simulink model "BLDCMachine_HystController_TorqueControl"  (R2018b)
settings: Solver=ode4  StartTime=0.0  StopTime=10  FixedStep=0.000005  MaxStep=1e-4  RelTol=1e-5
libraries: powerlib x16, dsparch4 x8, simulink x2
settings Model: Creator=uidp4945  LastModifiedBy=axint
settings SolverCC: AlgebraicLoopSolver=LineSearch
settings SFSimCC: SimUseLocalCustomCode=off
settings RTWCC: RTWUseLocalCustomCode=off

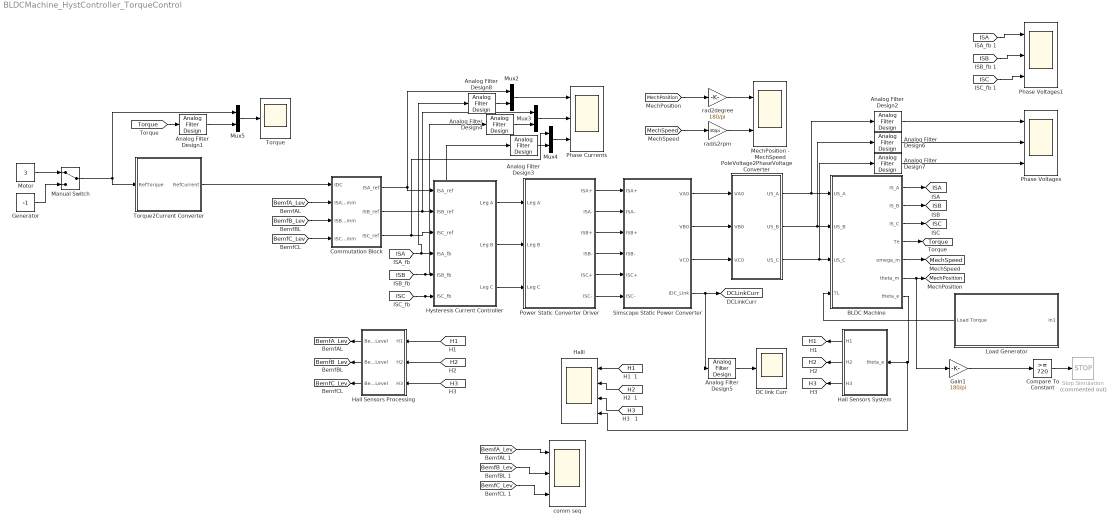
== system BLDCMachine_HystController_TorqueControl ==
  Analog Filter Design1 : dsparch4/Analog Filter Design  method=Butterworth  filttype=Lowpass  N=2  Wlo=500  Whi=80  Rp=2  Rs=40
  Analog Filter Design{2..8} (7 alike) : dsparch4/Analog Filter Design  method=Butterworth  filttype=Lowpass  N=2  Wlo=2000  Whi=80  Rp=2  Rs=40
  BLDC Machine : Subsystem  mask{Rs=0.2, Ls=0.0085*1e0, Flux=0.175, J=0.089, D=5e-5, p=4}
      mask prompts: Rs "Stator resistance [ohm]"; Ls "Equivalent stator inductance [H]"; Flux "Rotor magnetic flux [Wb]"; J "Moment of inertia [Kgm^2]"; D "Viscous coefficient [Nm s/rad]"; p "Number of pole pairs"
  Commutation Block : Subsystem
  Compare To Constant : simulink/Logic and Bit Operations/Compare To Constant  relop=>=  const=720  OutDataTypeStr=boolean
  DC link Curr : Scope
  Gain1 : Gain  Gain=180/pi
  Generator : Constant  Value=-1
  Hall Sensors Processing : Subsystem
  Hall Sensors System : Subsystem
  Halll : Scope  NumInputPorts=4
  Hysteresis Current Controller : Subsystem  mask{h=0.01}
      mask prompts: h "Hysteresis value [A]"
  Load Generator : Subsystem
  Manual Switch : ManualSwitch
  MechPosition - MechSpeed : Scope  NumInputPorts=2
  Motor : Constant  Value=3
  Mux{2..5} (4 alike) : Mux  Inputs=2
  Phase Currents : Scope  NumInputPorts=3
  Phase Voltages : Scope  NumInputPorts=3
  Phase Voltages1 : Scope  NumInputPorts=3
  PoleVoltage2PhaseVoltage Converter : Subsystem
  Power Static Converter Driver : Subsystem
  "Simscape Static Power Converter " : Subsystem  mask{VDC=500}
      mask prompts: VDC "Voltage DC Link"
  Stop Simulation : Stop  Commented=on
  "Torque " : Scope
  Torque2Current Converter : Subsystem  mask{Flux=0.175, p=4}
      mask prompts: Flux "Rotor Magnetic Flux [Wb]"; p "Number of pole pairs"
  comm seq : Scope  NumInputPorts=3
  rad/s2rpm : Gain  Gain=30/pi
  rad2degree : Gain  Gain=180/pi
  tag scope: BemfA_Lev=global, BemfB_Lev=global, BemfC_Lev=global, DCLinkCurr=global, H1=global, H2=global, H3=global, ISA=global, ISB=global, ISC=global, MechPosition=global, MechSpeed=global, Torque=global
  wires:
  "Simscape Static Power Converter "/1("VA0 ") -> PoleVoltage2PhaseVoltage Converter/1(VA0)
  "Simscape Static Power Converter "/2("VB0 ") -> PoleVoltage2PhaseVoltage Converter/2(VB0)
  "Simscape Static Power Converter "/3("VC0 ") -> PoleVoltage2PhaseVoltage Converter/3(VC0)
  PoleVoltage2PhaseVoltage Converter/1(US_A) -> Analog Filter Design2/1, BLDC Machine/1(US_A)
  PoleVoltage2PhaseVoltage Converter/2(US_B) -> Analog Filter Design6/1, BLDC Machine/2(US_B)
  PoleVoltage2PhaseVoltage Converter/3(US_C) -> Analog Filter Design7/1, BLDC Machine/3(US_C)
  Load Generator/1("Load Torque ") -> BLDC Machine/4(TL)
  BLDC Machine/1(IS_A) -> [ISA]
  BLDC Machine/2(IS_B) -> [ISB]
  BLDC Machine/3(IS_C) -> [ISC]
  BLDC Machine/5("omega_m  ") -> [MechSpeed]
  BLDC Machine/6("theta_m ") -> Gain1/1, [MechPosition]
  Hall Sensors System/1(H1) -> [H1]
  Hall Sensors System/2(H2) -> [H2]
  Hall Sensors System/3(H3) -> [H3]
  [H1] -> Hall Sensors Processing/1(H1)
  [H2] -> Hall Sensors Processing/2(H2)
  [H3] -> Hall Sensors Processing/3(H3)
  Hall Sensors Processing/1(BemfA Level) -> [BemfA_Lev]
  Hall Sensors Processing/2(BemfB Level) -> [BemfB_Lev]
  Hall Sensors Processing/3(BemfC Level) -> [BemfC_Lev]
  Power Static Converter Driver/2(ISA-) -> "Simscape Static Power Converter "/2(ISA-)
  Power Static Converter Driver/4(ISB-) -> "Simscape Static Power Converter "/4(ISB-)
  Power Static Converter Driver/6(ISC-) -> "Simscape Static Power Converter "/6(ISC-)
  Power Static Converter Driver/1(ISA+) -> "Simscape Static Power Converter "/1(ISA+)
  Power Static Converter Driver/3(ISB+) -> "Simscape Static Power Converter "/3(ISB+)
  Power Static Converter Driver/5(ISC+) -> "Simscape Static Power Converter "/5(ISC+)
  Hysteresis Current Controller/1(Leg A) -> Power Static Converter Driver/1(Leg A)
  Commutation Block/2(ISB_ref) -> Mux3/1, Hysteresis Current Controller/2(ISB_ref)
  Commutation Block/3(ISC_ref) -> Hysteresis Current Controller/3(ISC_ref), Mux4/1
  [ISB] -> Analog Filter Design4/1, Hysteresis Current Controller/5(ISB_fb)
  [ISC] -> Analog Filter Design3/1, Hysteresis Current Controller/6(ISC_fb)
  Hysteresis Current Controller/2(Leg B) -> Power Static Converter Driver/2(Leg B)
  Hysteresis Current Controller/3(Leg C) -> Power Static Converter Driver/3(Leg C)
  Mux2/1 -> Phase Currents/1
  Commutation Block/1(ISA_ref) -> Hysteresis Current Controller/1(ISA_ref), Mux2/1
  Mux3/1 -> Phase Currents/2
  Mux4/1 -> Phase Currents/3
  BLDC Machine/4(Te) -> [Torque]
  Mux5/1 -> "Torque "/1
  [Torque] -> Analog Filter Design1/1
  "Simscape Static Power Converter "/4(IDC_Link) -> Analog Filter Design5/1, [DCLinkCurr]
  [MechPosition] -> rad2degree/1
  [MechSpeed] -> rad/s2rpm/1
  rad2degree/1 -> MechPosition - MechSpeed/1
  rad/s2rpm/1 -> MechPosition - MechSpeed/2
  Analog Filter Design1/1 -> Mux5/2
  Torque2Current Converter/1(RefCurrent) -> Commutation Block/1(IDC)
  Analog Filter Design2/1 -> Phase Voltages/1
  Manual Switch/1 -> Mux5/1, Torque2Current Converter/1(RefTorque)
  Analog Filter Design3/1 -> Mux4/2
  Analog Filter Design4/1 -> Mux3/2
  Analog Filter Design6/1 -> Phase Voltages/2
  Analog Filter Design7/1 -> Phase Voltages/3
  [ISA] -> Analog Filter Design8/1, Hysteresis Current Controller/4(ISA_fb)
  [BemfA_Lev] -> Commutation Block/2(ISA comm)
  [BemfB_Lev] -> Commutation Block/3(ISB comm)
  [BemfC_Lev] -> Commutation Block/4(ISC comm)
  Gain1/1 -> Compare To Constant/1
  Compare To Constant/1 -> Stop Simulation/1
  Generator/1 -> Manual Switch/2
  Motor/1 -> Manual Switch/1
  Analog Filter Design5/1 -> DC link Curr/1
  [H1] -> Halll/1
  [H2] -> Halll/2
  [H3] -> Halll/3
  BLDC Machine/7(theta_e) -> Halll/4, Hall Sensors System/1(theta_e)
  [ISA] -> Phase Voltages1/1
  [ISB] -> Phase Voltages1/2
  [ISC] -> Phase Voltages1/3
  Analog Filter Design8/1 -> Mux2/2
  [BemfA_Lev] -> comm seq/1
  [BemfB_Lev] -> comm seq/2
  [BemfC_Lev] -> comm seq/3

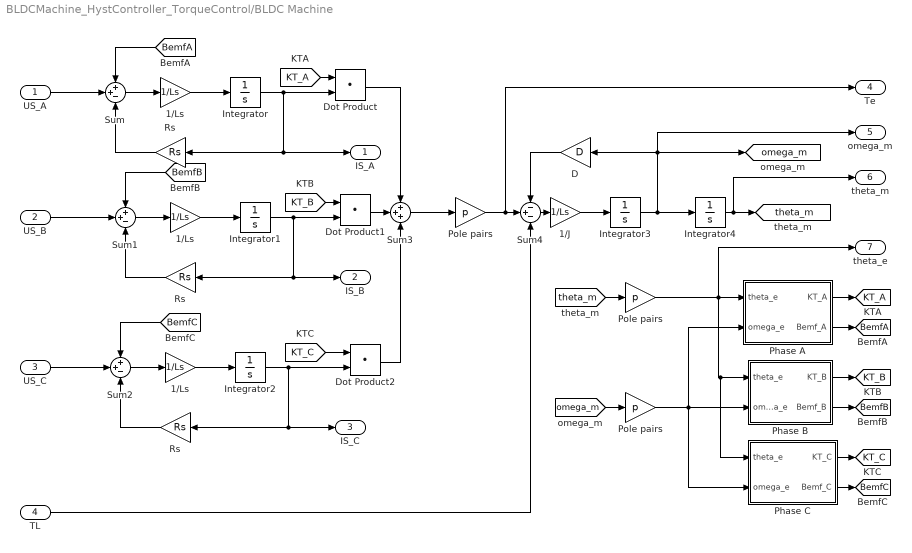
== system BLDCMachine_HystController_TorqueControl/BLDC Machine ==
  US_A : Inport
  US_B : Inport  Port=2
  US_C : Inport  Port=3
  TL : Inport  Port=4
  1/J : Gain  Gain=1/Ls
  1/Ls : Gain  Gain=1/Ls
  "1/Ls " : Gain  Gain=1/Ls
  "1/Ls  " : Gain  Gain=1/Ls
  D : Gain  Gain=D
  Dot Product : DotProduct  InputSameDT=on  OutDataTypeStr=Inherit: Inherit via internal rule
  Dot Product1 : DotProduct  InputSameDT=on  OutDataTypeStr=Inherit: Inherit via internal rule
  Dot Product2 : DotProduct  InputSameDT=on  OutDataTypeStr=Inherit: Inherit via internal rule
  Integrator{,1..4} (5 alike) : Integrator
  Phase A : Subsystem
  Phase B : Subsystem
  Phase C : Subsystem
  Pole pairs : Gain  Gain=p
  "Pole pairs  " : Gain  Gain=p
  "Pole pairs   " : Gain  Gain=p
  Rs : Gain  Gain=Rs
  "Rs " : Gain  Gain=Rs
  "Rs  " : Gain  Gain=Rs
  Sum : Sum  Inputs=++-
  Sum1 : Sum  Inputs=++-
  Sum2 : Sum  Inputs=++-
  Sum3 : Sum  Inputs=+++
  Sum4 : Sum  Inputs=-+-
  IS_A : Outport
  IS_B : Outport  Port=2
  IS_C : Outport  Port=3
  Te : Outport  Port=4
  "omega_m  " : Outport  Port=5
  "theta_m " : Outport  Port=6
  theta_e : Outport  Port=7
  tag scope: BemfA=global, BemfB=global, BemfC=global, KT_A=global, KT_B=global, KT_C=global, omega_m=global, theta_m=global
  wires:
  [KT_C] -> Dot Product2/1
  Sum4/1 -> 1/J/1
  Dot Product1/1 -> Sum3/2
  Phase B/1(KT_B) -> [KT_B]
  Phase A/1(KT_A) -> [KT_A]
  Dot Product2/1 -> Sum3/3
  Dot Product/1 -> Sum3/1
  Phase C/1(KT_C) -> [KT_C]
  Integrator/1 -> Dot Product/2, IS_A/1, Rs/1
  Integrator4/1 -> [theta_m], "theta_m "/1
  Pole pairs/1 -> Phase C/2(omega_e), Phase B/2(omega_e), Phase A/2(omega_e)
  "Pole pairs  "/1 -> theta_e/1, Phase C/1(theta_e), Phase B/1(theta_e), Phase A/1(theta_e)
  D/1 -> Sum4/1
  [BemfC] -> Sum2/1
  Sum2/1 -> "1/Ls  "/1
  "1/Ls  "/1 -> Integrator2/1
  Integrator2/1 -> Dot Product2/2, IS_C/1, "Rs  "/1
  US_C/1 -> Sum2/2
  "Rs  "/1 -> Sum2/3
  Phase B/2(Bemf_B) -> [BemfB]
  Phase C/2(Bemf_C) -> [BemfC]
  Integrator1/1 -> Dot Product1/2, IS_B/1, "Rs "/1
  1/J/1 -> Integrator3/1
  [omega_m] -> Pole pairs/1
  [KT_B] -> Dot Product1/1
  Phase A/2(Bemf_A) -> [BemfA]
  TL/1 -> Sum4/3
  [KT_A] -> Dot Product/1
  [BemfA] -> Sum/1
  US_A/1 -> Sum/2
  Rs/1 -> Sum/3
  [theta_m] -> "Pole pairs  "/1
  Integrator3/1 -> "omega_m  "/1, D/1, [omega_m], Integrator4/1
  1/Ls/1 -> Integrator/1
  "1/Ls "/1 -> Integrator1/1
  Sum1/1 -> "1/Ls "/1
  US_B/1 -> Sum1/2
  "Rs "/1 -> Sum1/3
  [BemfB] -> Sum1/1
  Sum/1 -> 1/Ls/1
  Sum3/1 -> "Pole pairs   "/1
  "Pole pairs   "/1 -> Te/1, Sum4/2

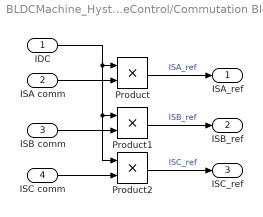
== system BLDCMachine_HystController_TorqueControl/Commutation Block ==
  IDC : Inport
  ISA comm : Inport  Port=2
  ISB comm : Inport  Port=3
  ISC comm : Inport  Port=4
  Product : Product
  Product1 : Product
  Product2 : Product
  ISA_ref : Outport
  ISB_ref : Outport  Port=2
  ISC_ref : Outport  Port=3
  wires:
  ISC comm/1 -> Product2/2
  Product/1 -> ISA_ref/1  "ISA_ref"
  IDC/1 -> Product2/1, Product1/1, Product/1
  ISB comm/1 -> Product1/2
  ISA comm/1 -> Product/2
  Product2/1 -> ISC_ref/1  "ISC_ref"
  Product1/1 -> ISB_ref/1  "ISB_ref"

== system BLDCMachine_HystController_TorqueControl/Hall Sensors Processing ==
  H1 : Inport
  H2 : Inport  Port=2
  H3 : Inport  Port=3
  BemfA Saturation Level : Subsystem
  BemfB Saturation Level : Subsystem
  BemfC Saturation Level : Subsystem
  BemfA Level : Outport
  BemfB Level : Outport  Port=2
  BemfC Level : Outport  Port=3
  wires:
  BemfB Saturation Level/1("BenfB Level ") -> BemfB Level/1
  H2/1 -> BemfC Saturation Level/1(H2), BemfB Saturation Level/2(H2)
  H1/1 -> BemfB Saturation Level/1(H1), BemfA Saturation Level/1(H1)
  BemfC Saturation Level/1("BenfC Level ") -> BemfC Level/1
  BemfA Saturation Level/1("BenfA Level ") -> BemfA Level/1
  H3/1 -> BemfC Saturation Level/2(H3), BemfA Saturation Level/2(H3)

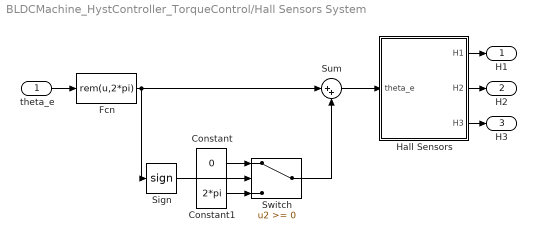
== system BLDCMachine_HystController_TorqueControl/Hall Sensors System ==
  theta_e : Inport
  Constant : Constant  Value=0
  Constant1 : Constant  Value=2*pi
  Fcn : Fcn  Expr=rem(u,2*pi)
  Hall Sensors : Subsystem
  Sign : Signum
  Sum : Sum  Inputs=|++
  Switch : Switch
  H1 : Outport
  H2 : Outport  Port=2
  H3 : Outport  Port=3
  wires:
  Hall Sensors/3("H3 ") -> H3/1
  Hall Sensors/1("H1 ") -> H1/1
  Hall Sensors/2("H2 ") -> H2/1
  theta_e/1 -> Fcn/1
  Fcn/1 -> Sum/1, Sign/1
  Sign/1 -> Switch/2
  Constant1/1 -> Switch/3
  Switch/1 -> Sum/2
  Sum/1 -> Hall Sensors/1(theta_e)
  Constant/1 -> Switch/1

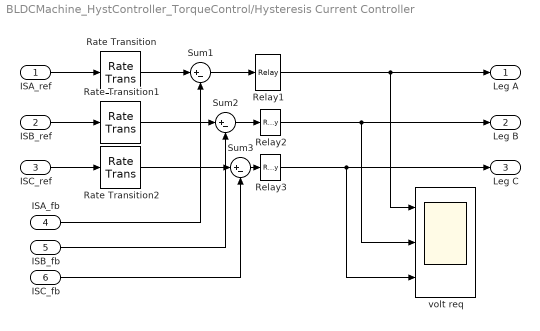
== system BLDCMachine_HystController_TorqueControl/Hysteresis Current Controller ==
  ISA_ref : Inport
  ISB_ref : Inport  Port=2
  ISC_ref : Inport  Port=3
  ISA_fb : Inport  Port=4
  ISB_fb : Inport  Port=5
  ISC_fb : Inport  Port=6
  Rate Transition : RateTransition  OutPortSampleTime=0.000025
  Rate Transition1 : RateTransition  OutPortSampleTime=0.000025
  Rate Transition2 : RateTransition  OutPortSampleTime=0.000025
  Relay1 : Relay  OnSwitchValue=h/2  OffSwitchValue=-h/2  OffOutputValue=-1
  Relay2 : Relay  OnSwitchValue=h/2  OffSwitchValue=-h/2  OffOutputValue=-1
  Relay3 : Relay  OnSwitchValue=h/2  OffSwitchValue=-h/2  OffOutputValue=-1
  Sum1 : Sum  Inputs=|+-
  Sum2 : Sum  Inputs=|+-
  Sum3 : Sum  Inputs=|+-
  volt req : Scope  NumInputPorts=3
  Leg A : Outport
  Leg B : Outport  Port=2
  Leg C : Outport  Port=3
  wires:
  ISC_fb/1 -> Sum3/2
  ISA_fb/1 -> Sum1/2
  Sum3/1 -> Relay3/1
  ISA_ref/1 -> Rate Transition/1
  Sum2/1 -> Relay2/1
  ISB_fb/1 -> Sum2/2
  Relay1/1 -> volt req/1, Leg A/1
  Relay2/1 -> volt req/2, Leg B/1
  Sum1/1 -> Relay1/1
  ISC_ref/1 -> Rate Transition2/1
  Relay3/1 -> volt req/3, Leg C/1
  ISB_ref/1 -> Rate Transition1/1
  Rate Transition/1 -> Sum1/1
  Rate Transition1/1 -> Sum2/1
  Rate Transition2/1 -> Sum3/1

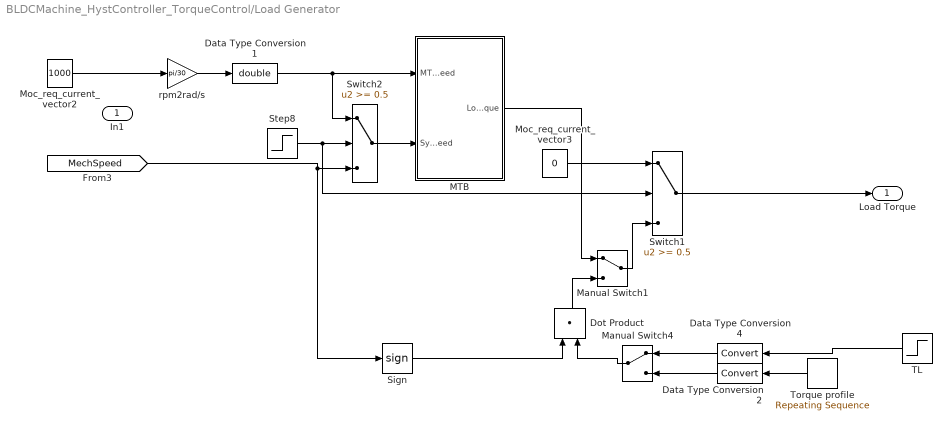
== system BLDCMachine_HystController_TorqueControl/Load Generator ==
  In1 : Inport
  Data Type Conversion1 : DataTypeConversion  OutDataTypeStr=double
  Data Type Conversion2 : DataTypeConversion
  Data Type Conversion4 : DataTypeConversion
  Dot Product : DotProduct  InputSameDT=on  OutDataTypeStr=Inherit: Inherit via internal rule
  MTB : Subsystem
  Manual Switch1 : ManualSwitch
  Manual Switch4 : ManualSwitch
  Moc_req_current_vector2 : Constant  Value=1000  OutDataTypeStr=Inherit: Inherit via back propagation
  Moc_req_current_vector3 : Constant  Value=0  OutDataTypeStr=Inherit: Inherit via back propagation
  Sign : Signum
  Step8 : Step  Time=0  Before=1  After=0  SampleTime=0
  Switch1 : Switch  Threshold=0.5
  Switch2 : Switch  Threshold=0.5
  TL : Step  Time=0.5  After=10*0.5  SampleTime=0
  Torque profile : simulink/Sources/Repeating Sequence  rep_seq_t="[0 0.12    0.24   0.48 ]"  rep_seq_y="[1   1     -1 -1]*0"
  rpm2rad/s : Gain  Gain=pi/30
  "Load Torque " : Outport
  wires:
  Switch2/1 -> MTB/2(Sys_Speed)
  Manual Switch1/1 -> Switch1/3
  Step8/1 -> Switch1/2, Switch2/2
  MTB/1(Load_Torque) -> Manual Switch1/1
  Moc_req_current_vector3/1 -> Switch1/1
  Dot Product/1 -> Manual Switch1/2
  Sign/1 -> Dot Product/1
  Manual Switch4/1 -> Dot Product/2
  Torque profile/1 -> Data Type Conversion2/1
  Data Type Conversion2/1 -> Manual Switch4/2
  Data Type Conversion4/1 -> Manual Switch4/1
  Moc_req_current_vector2/1 -> rpm2rad/s/1
  Data Type Conversion1/1 -> Switch2/1, MTB/1(MTB_Speed)
  TL/1 -> Data Type Conversion4/1
  rpm2rad/s/1 -> Data Type Conversion1/1
  [MechSpeed] -> Switch2/3, Sign/1
  Switch1/1 -> "Load Torque "/1

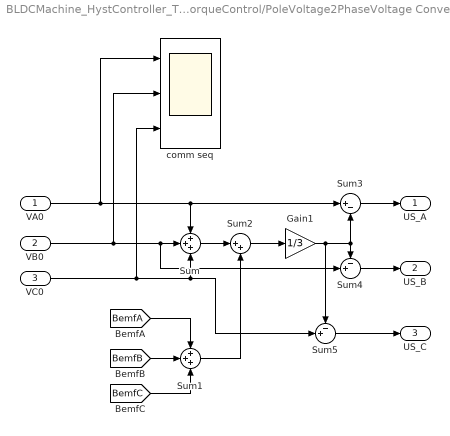
== system BLDCMachine_HystController_TorqueControl/PoleVoltage2PhaseVoltage Converter ==
  VA0 : Inport
  VB0 : Inport  Port=2
  VC0 : Inport  Port=3
  Gain1 : Gain  Gain=1/3
  Sum : Sum  Inputs=+++
  Sum1 : Sum  Inputs=+++
  Sum2 : Sum  Inputs=|++
  Sum3 : Sum  Inputs=|+-
  Sum4 : Sum  Inputs=-+|
  Sum5 : Sum  Inputs=-+|
  comm seq : Scope  NumInputPorts=3
  US_A : Outport
  US_B : Outport  Port=2
  US_C : Outport  Port=3
  wires:
  VB0/1 -> comm seq/2, Sum4/2, Sum/2
  [BemfC] -> Sum1/3
  [BemfA] -> Sum1/1
  [BemfB] -> Sum1/2
  VC0/1 -> comm seq/3, Sum5/2, Sum/3
  Sum3/1 -> US_A/1
  VA0/1 -> comm seq/1, Sum3/1, Sum/1
  Sum1/1 -> Sum2/2
  Sum4/1 -> US_B/1
  Sum/1 -> Sum2/1
  Sum2/1 -> Gain1/1
  Gain1/1 -> Sum4/1, Sum3/2, Sum5/1
  Sum5/1 -> US_C/1

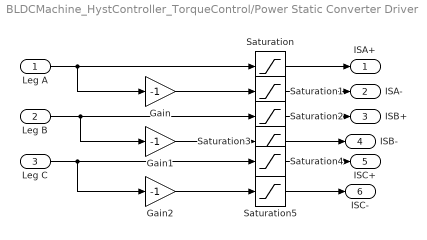
== system BLDCMachine_HystController_TorqueControl/Power Static Converter Driver ==
  Leg A : Inport
  Leg B : Inport  Port=2
  Leg C : Inport  Port=3
  Gain : Gain  Gain=-1
  Gain1 : Gain  Gain=-1
  Gain2 : Gain  Gain=-1
  Saturation{,1..5} (6 alike) : Saturate  UpperLimit=1  LowerLimit=0
  ISA+ : Outport
  ISA- : Outport  Port=2
  ISB+ : Outport  Port=3
  ISB- : Outport  Port=4
  ISC+ : Outport  Port=5
  ISC- : Outport  Port=6
  wires:
  Gain/1 -> Saturation1/1
  Gain1/1 -> Saturation3/1
  Leg C/1 -> Gain2/1, Saturation4/1
  Leg A/1 -> Gain/1, Saturation/1
  Gain2/1 -> Saturation5/1
  Leg B/1 -> Gain1/1, Saturation2/1
  Saturation/1 -> ISA+/1
  Saturation1/1 -> ISA-/1
  Saturation2/1 -> ISB+/1
  Saturation3/1 -> ISB-/1
  Saturation4/1 -> ISC+/1
  Saturation5/1 -> ISC-/1

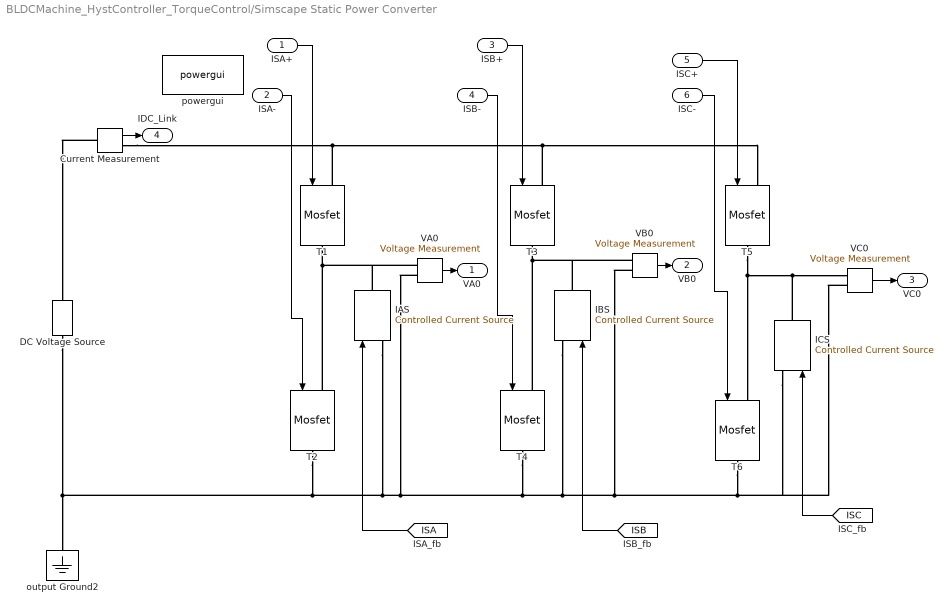
== system BLDCMachine_HystController_TorqueControl/Simscape Static Power Converter  ==
  ISA+ : Inport
  ISA- : Inport  Port=2
  ISB+ : Inport  Port=3
  ISB- : Inport  Port=4
  ISC+ : Inport  Port=5
  ISC- : Inport  Port=6
  Current Measurement : powerlib/Measurements/Current Measurement  PhasorSimulation=off  OutputType=Complex  PSBequivalent=0
      settings: SourceProductName=Simscape Electrical
  DC Voltage Source : powerlib/Electrical Sources/DC Voltage Source  Amplitude=VDC  Measurements=None
      settings: SourceProductName=Simscape Electrical
  IAS : powerlib/Electrical Sources/Controlled Current Source  Initialize=on  Source_Type=DC  Amplitude=0  Phase=0  Frequency=0  Measurements=None
      settings: SourceProductName=Simscape Electrical
  IBS : powerlib/Electrical Sources/Controlled Current Source  Initialize=on  Source_Type=DC  Amplitude=0  Phase=0  Frequency=0  Measurements=None
      settings: SourceProductName=Simscape Electrical
  ICS : powerlib/Electrical Sources/Controlled Current Source  Initialize=on  Source_Type=DC  Amplitude=0  Phase=0  Frequency=0  Measurements=None
      settings: SourceProductName=Simscape Electrical
  T{1..6} (6 alike) : powerlib/Power Electronics/Mosfet  Ron=0.1  Lon=0  Rd=0.01  Vfd=0  IC=0  Rs=1e5  Cs=inf  Measurements=off
      settings: SourceProductName=Simscape Electrical
  VA0 : powerlib/Measurements/Voltage Measurement  PhasorSimulation=off  OutputType=Complex  PSBequivalent=0
      settings: SourceProductName=Simscape Electrical
  VB0 : powerlib/Measurements/Voltage Measurement  PhasorSimulation=off  OutputType=Complex  PSBequivalent=0
      settings: SourceProductName=Simscape Electrical
  VC0 : powerlib/Measurements/Voltage Measurement  PhasorSimulation=off  OutputType=Complex  PSBequivalent=0
      settings: SourceProductName=Simscape Electrical
  output Ground2 : powerlib/Elements/Ground  LConnTagsString=a
      settings: SourceProductName=Simscape Electrical
  powergui : powerlib/powergui  Priority=1  SimulationMode=Continuous  SampleTime=0.0001  frequency=60  Iterations=50  frequencyindice=0  Pbase=100e6  ErrMax=1e-4  UnitsV=kV  UnitsW=MW  buscounter=0  FunctionMessages=off  echomessages=off  EnableUseOfTLC=off  CurrentSourceSwitches=off  DisableSnubberDevices=off  DisableRonSwitches=off  DisableVfSwitches=off  DisplayEquations=off  SolverType=Tustin/Backward Euler (TBE)  Interpol=off  ExternalGateDelay=off  methode=off  Ts=100  x0status=blocks  SPID=on  SwTol=0  HookPort=off  RestoreLinks=warning  ResistiveCurrentMeasurement=off  Frange=[0:2:500]  Ylog=off  Xlog=on  ShowGrid=off  save=off  variable=ZData  structure=0  ZoomFFT=off  StartTime=0.0  cycles=1  DisplayStyle=1  fundamental=60  FreqAxis=off  MaxFrequency=1000  frequencyindicesteady=1  RmsSteady=1  display=off
  "VA0 " : Outport
  "VB0 " : Outport  Port=2
  "VC0 " : Outport  Port=3
  IDC_Link : Outport  Port=4
  wires:
  Current Measurement/1 -> IDC_Link/1
  VC0/1 -> "VC0 "/1
  VA0/1 -> "VA0 "/1
  VB0/1 -> "VB0 "/1
  ISC+/1 -> T5/1
  ISC-/1 -> T6/1
  ISB+/1 -> T3/1
  ISA+/1 -> T1/1
  ISA-/1 -> T2/1
  ISB-/1 -> T4/1
  [ISA] -> IAS/1
  [ISB] -> IBS/1
  [ISC] -> ICS/1
  connections:
  DC Voltage Source/LConn1 -- IAS/LConn1 -- IBS/LConn1 -- ICS/LConn1 -- VC0/LConn2 -- T6/RConn1 -- VB0/LConn2 -- T4/RConn1 -- VA0/LConn2 -- T2/RConn1 -- output Ground2/LConn1
  Current Measurement/RConn1 -- T1/LConn1 -- T5/LConn1 -- T3/LConn1
  Current Measurement/LConn1 -- DC Voltage Source/RConn1
  T5/RConn1 -- ICS/RConn1 -- VC0/LConn1 -- T6/LConn1
  T4/LConn1 -- IBS/RConn1 -- VB0/LConn1 -- T3/RConn1
  T2/LConn1 -- IAS/RConn1 -- VA0/LConn1 -- T1/RConn1

== system BLDCMachine_HystController_TorqueControl/Torque2Current Converter ==
  RefTorque : Inport
  torque2current : Gain  Gain=1/(2*p*Flux)
  RefCurrent : Outport
  wires:
  torque2current/1 -> RefCurrent/1
  RefTorque/1 -> torque2current/1

== system BLDCMachine_HystController_TorqueControl/BLDC Machine/Phase A ==
  theta_e : Inport
  omega_e : Inport  Port=2
  Fcn : Fcn
  Fcn1 : Fcn  Expr=rem(u,2*pi)
  KE/KT : Gain  Gain=Flux/0.5  SaturateOnIntegerOverflow=on  OutDataTypeStr=Inherit: Same as input  ParamDataTypeStr=Inherit: Same as input
  Product1 : Product  SaturateOnIntegerOverflow=on  OutDataTypeStr=Inherit: Same as first input
  Saturation : Saturate
  KT_A : Outport
  Bemf_A : Outport  Port=2
  wires:
  Fcn/1 -> Saturation/1
  Saturation/1 -> KE/KT/1
  omega_e/1 -> Product1/2
  Product1/1 -> Bemf_A/1
  theta_e/1 -> Fcn1/1
  Fcn1/1 -> Fcn/1
  KE/KT/1 -> KT_A/1, Product1/1

== system BLDCMachine_HystController_TorqueControl/BLDC Machine/Phase B ==
  theta_e : Inport
  omega_e : Inport  Port=2
  Fcn : Fcn  Expr=sin(u[1]-2*pi/3)
  Fcn1 : Fcn  Expr=rem(u,2*pi)
  Gain4 : Gain  Gain=Flux/0.5  SaturateOnIntegerOverflow=on  OutDataTypeStr=Inherit: Same as input  ParamDataTypeStr=Inherit: Same as input
  Product1 : Product  SaturateOnIntegerOverflow=on  OutDataTypeStr=Inherit: Same as first input
  Saturation : Saturate
  KT_B : Outport
  Bemf_B : Outport  Port=2
  wires:
  Saturation/1 -> Gain4/1
  omega_e/1 -> Product1/2
  theta_e/1 -> Fcn1/1
  Fcn/1 -> Saturation/1
  Product1/1 -> Bemf_B/1
  Fcn1/1 -> Fcn/1
  Gain4/1 -> KT_B/1, Product1/1

== system BLDCMachine_HystController_TorqueControl/BLDC Machine/Phase C ==
  theta_e : Inport
  omega_e : Inport  Port=2
  Fcn : Fcn  Expr=sin(u[1]+2*pi/3)
  Fcn1 : Fcn  Expr=rem(u,2*pi)
  Gain4 : Gain  Gain=Flux/0.5  SaturateOnIntegerOverflow=on  OutDataTypeStr=Inherit: Same as input  ParamDataTypeStr=Inherit: Same as input
  Product1 : Product  SaturateOnIntegerOverflow=on  OutDataTypeStr=Inherit: Same as first input
  Saturation : Saturate
  KT_C : Outport
  Bemf_C : Outport  Port=2
  wires:
  Product1/1 -> Bemf_C/1
  omega_e/1 -> Product1/2
  Fcn/1 -> Saturation/1
  theta_e/1 -> Fcn1/1
  Saturation/1 -> Gain4/1
  Fcn1/1 -> Fcn/1
  Gain4/1 -> KT_C/1, Product1/1

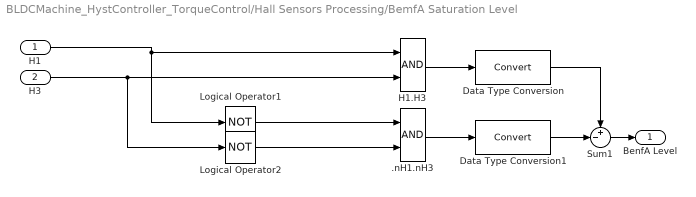
== system BLDCMachine_HystController_TorqueControl/Hall Sensors Processing/BemfA Saturation Level ==
  H1 : Inport
  H3 : Inport  Port=2
  .nH1.nH3 : Logic  AllPortsSameDT=off  OutDataTypeStr=boolean
  Data Type Conversion : DataTypeConversion
  Data Type Conversion1 : DataTypeConversion
  "H1.H3 " : Logic  AllPortsSameDT=off  OutDataTypeStr=boolean
  Logical Operator1 : Logic  Operator=NOT  AllPortsSameDT=off  OutDataTypeStr=boolean
  Logical Operator2 : Logic  Operator=NOT  AllPortsSameDT=off  OutDataTypeStr=boolean
  Sum1 : Sum  Inputs=+-|
  "BenfA Level " : Outport
  wires:
  H1/1 -> Logical Operator1/1, "H1.H3 "/1
  H3/1 -> "H1.H3 "/2, Logical Operator2/1
  Logical Operator1/1 -> .nH1.nH3/1
  Sum1/1 -> "BenfA Level "/1
  Data Type Conversion1/1 -> Sum1/2
  Data Type Conversion/1 -> Sum1/1
  "H1.H3 "/1 -> Data Type Conversion/1
  .nH1.nH3/1 -> Data Type Conversion1/1
  Logical Operator2/1 -> .nH1.nH3/2

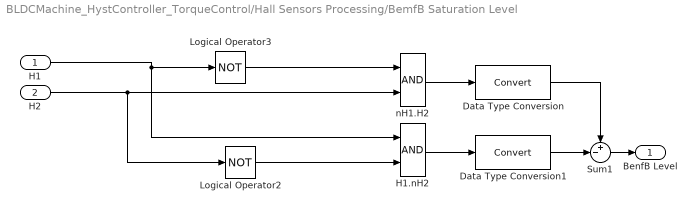
== system BLDCMachine_HystController_TorqueControl/Hall Sensors Processing/BemfB Saturation Level ==
  H1 : Inport
  H2 : Inport  Port=2
  Data Type Conversion : DataTypeConversion
  Data Type Conversion1 : DataTypeConversion
  H1.nH2 : Logic  AllPortsSameDT=off  OutDataTypeStr=boolean
  Logical Operator2 : Logic  Operator=NOT  AllPortsSameDT=off  OutDataTypeStr=boolean
  Logical Operator3 : Logic  Operator=NOT  AllPortsSameDT=off  OutDataTypeStr=boolean
  Sum1 : Sum  Inputs=+-|
  "nH1.H2 " : Logic  AllPortsSameDT=off  OutDataTypeStr=boolean
  "BenfB Level " : Outport
  wires:
  Logical Operator2/1 -> H1.nH2/2
  H1.nH2/1 -> Data Type Conversion1/1
  "nH1.H2 "/1 -> Data Type Conversion/1
  Data Type Conversion/1 -> Sum1/1
  Data Type Conversion1/1 -> Sum1/2
  Sum1/1 -> "BenfB Level "/1
  H1/1 -> H1.nH2/1, Logical Operator3/1
  H2/1 -> Logical Operator2/1, "nH1.H2 "/2
  Logical Operator3/1 -> "nH1.H2 "/1

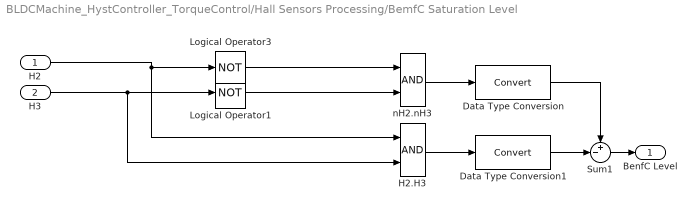
== system BLDCMachine_HystController_TorqueControl/Hall Sensors Processing/BemfC Saturation Level ==
  H2 : Inport
  H3 : Inport  Port=2
  Data Type Conversion : DataTypeConversion
  Data Type Conversion1 : DataTypeConversion
  H2.H3 : Logic  AllPortsSameDT=off  OutDataTypeStr=boolean
  Logical Operator1 : Logic  Operator=NOT  AllPortsSameDT=off  OutDataTypeStr=boolean
  Logical Operator3 : Logic  Operator=NOT  AllPortsSameDT=off  OutDataTypeStr=boolean
  Sum1 : Sum  Inputs=+-|
  "nH2.nH3 " : Logic  AllPortsSameDT=off  OutDataTypeStr=boolean
  "BenfC Level " : Outport
  wires:
  Logical Operator3/1 -> "nH2.nH3 "/1
  H2/1 -> Logical Operator3/1, H2.H3/1
  Sum1/1 -> "BenfC Level "/1
  Data Type Conversion1/1 -> Sum1/2
  Data Type Conversion/1 -> Sum1/1
  "nH2.nH3 "/1 -> Data Type Conversion/1
  H2.H3/1 -> Data Type Conversion1/1
  H3/1 -> H2.H3/2, Logical Operator1/1
  Logical Operator1/1 -> "nH2.nH3 "/2

== system BLDCMachine_HystController_TorqueControl/Hall Sensors System/Hall Sensors ==
  theta_e : Inport
  H1 : Fcn  Expr=(u>=0 && u<=5*pi/6) || (u>=11*pi/6 && u<=2*pi)
  H2 : Fcn  Expr=u>=pi/2 && u<=3*pi/2
  H3 : Fcn  Expr=(u>=pi/6 && u<=7*pi/6)
  "H1 " : Outport
  "H2 " : Outport  Port=2
  "H3 " : Outport  Port=3
  wires:
  theta_e/1 -> H3/1, H1/1, H2/1
  H1/1 -> "H1 "/1
  H2/1 -> "H2 "/1
  H3/1 -> "H3 "/1

== system BLDCMachine_HystController_TorqueControl/Load Generator/MTB ==
  MTB_Speed : Inport
  Sys_Speed : Inport  Port=2
  Gain : Gain  Gain=-0.2
  PI_q1 : Subsystem
  Saturation2 : Saturate  UpperLimit=100  LowerLimit=-100
  Sum1 : Sum  Inputs=+|-
  Sum2 : Sum  Inputs=|+-
  Load_Torque : Outport
  wires:
  MTB_Speed/1 -> Sum2/1
  Sys_Speed/1 -> Sum2/2
  PI_q1/1(u) -> Gain/1
  Sum2/1 -> PI_q1/1(e)
  Gain/1 -> Saturation2/1, Sum1/1
  Sum1/1 -> PI_q1/2(anti Wup)
  Saturation2/1 -> Sum1/2, Load_Torque/1

== system BLDCMachine_HystController_TorqueControl/Load Generator/MTB/PI_q1 ==
  e : Inport
  anti Wup : Inport  Port=2
  Gain : Gain  Gain=400
  Gain1 : Gain  Gain=800
  Gain2 : Gain  Gain=20
  Integrator : Integrator
  Sum : Sum  Inputs=|++
  Sum1 : Sum  Inputs=|+-
  u : Outport
  wires:
  e/1 -> Gain/1, Gain1/1
  Sum/1 -> u/1
  Integrator/1 -> Sum/2
  Gain1/1 -> Sum/1
  Sum1/1 -> Integrator/1
  Gain/1 -> Sum1/1
  Gain2/1 -> Sum1/2
  anti Wup/1 -> Gain2/1
